simulink model "ppfx"  (Simulink 3.00)
settings: Solver=ode45  StartTime=0.0  StopTime=40  MaxStep=0.01  RelTol=1e-3  AbsTol=1e-3
undefined symbols (not defined in the file): offset, ssfunpsd
settings Model: SaveTime=off  SaveOutput=off

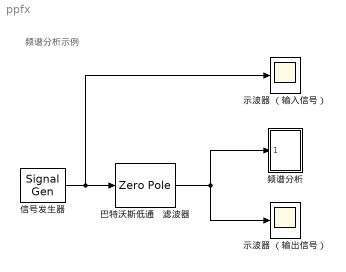
== system ppfx ==
  note: 频谱分析示例
  "  巴特沃斯低通   滤波器" : ZeroPole  Zeros=z  Poles=p  Gain=k  mask(buttap){@1=200, @2=4}
      mask prompts: @1 "Cutoff frequency (rad/sec)"; @2 "Order"
      mask help:
      | Analog Butterworth low pass filter.
      |
      | (Requires Signal Processing Toolbox)
      mask init:
      | [z,p,k]=buttap(@2); z=@1*z; p=@1*p; k=real(prod(-p)); [num,den]=zp2tf(z,p,k); w=logspace(log10(@1/10),log10(10*@1),20); h=freqs(num,den,w);
      mask Help: Butterworth low pass filter using MATLAB's butter command.
      mask Display: plot(20*log10(w),20*log10(abs(h)))
  频谱分析 : Subsystem  LoadFcn=ssfunpsd([],[],[],'LoadBlock')  StartFcn=ssfunpsd([],[],[],'Start')  mask(Spectrum analyzer.){@1=256, @2=512, @3=64, @4=0.1}
      mask prompts: @1 "Length of buffer:"; @2 "Number of points for fft:"; @3 "Plot after how many points:"; @4 "Sample time:"
      mask help: Spectrum analyser using graph window.
      mask init:
      | npts=@1; fftpts=@2; HowOften=@3; ts=@4(1); if length(@4) > 1, offset = @4(2), else, offset = 0; end
      settings: CopyFcn=ssfunpsd([],[],[],'CopyBlock')  DeleteFcn=ssfunpsd([],[],[],'DeleteBlock')  NameChangeFcn=ssfunpsd([],[],[],'NameChange')
      mask Help: This block when hooked to the output of a system displays the frequency content of the buffer in the graph window. For more see the M-file specanal.
      mask Display: plot(0,0,100,100,[14,91,91,14,14],[86,86,40,40,86],[85,82,80,79,75,67,63,60,57,53,41,36,33,27,24],[49,50,53,50,49,51,54,66,54,50,50,52,81,51,49])
  示波器 （输出信号） : Scope
      settings: TimeRange=30.000000  YMin=-1.5  YMax=1.5  SaveToWorkspace=off  SaveName=ScopeData  DataFormat=Matrix
  示波器 （输入信号） : Scope
      settings: TimeRange=30.000000  YMin=-1.5  YMax=1.5  SaveToWorkspace=off  SaveName=ScopeData  DataFormat=Matrix
  信号发生器 : SignalGenerator  WaveForm=square  Amplitude=1.000000  Frequency=5.000000  Units=rad/sec
  wires:
  "  巴特沃斯低通   滤波器"/1 -> 频谱分析/1(input signal), 示波器 （输出信号）/1
  信号发生器/1 -> "  巴特沃斯低通   滤波器"/1, 示波器 （输入信号）/1

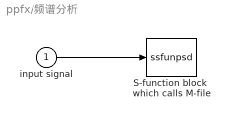
== system ppfx/频谱分析 ==
  input signal : Inport  Port=1  PortWidth=-1  SampleTime=-1  DataType=auto
      settings: SignalType=auto
  S-function block  which calls M-file : S-Function  FunctionName=ssfunpsd  Parameters=fftpts,npts,HowOften,offset,ts,0  PortCounts=[]  SFunctionModules=''
  wires:
  input signal/1 -> S-function block  which calls M-file/1
